simulink model "sgMdl_IO207_DigitalLoopback"  (R2024b)
settings: Solver=FixedStepAuto  StartTime=0.0  StopTime=inf  RelTol=1e-3
undefined symbols (not defined in the file): IO1, IO128, IO64, IO65
libraries: speedgoatlib_IO207 x5
Description:
  | IO207 - Digital Loopback
settings Model: ModifiedByFormat=Speedgoat  Creator=Speedgoat  LastModifiedBy=Speedgoat
settings SolverCC: ConcurrentTasks=on  AlgebraicLoopSolver=TrustRegion  PositivePriorityOrder=on
settings DataIOCC: LimitDataPoints=on  SaveFormat=Array  ReturnWorkspaceOutputs=off
settings OptimizationCC: BlockReduction=off  OptimizeBlockIOStorage=off  BufferReuse=off  ReuseModelBlockBuffer=off  GlobalBufferReuse=off  ExpressionFolding=off  ExpressionDepthLimit=2147483647  LocalBlockOutputs=off  OptimizeDataStoreBuffers=off  BusAssignmentInplaceUpdate=off
settings DebuggingCC: UnderspecifiedInitializationDetection=Classic  MergeDetectMultiDrivingBlocksExec=none  SolverPrmCheckMsg=warning  TasksWithSamePriorityMsg=none  FcnCallInpInsideContextMsg=warning  StateNameClashWarn=warning  SFUnexpectedBacktrackingDiag=warning  SFNoUnconditionalDefaultTransitionDiag=warning  SFExecutionAtInitializationDiag=none  ArithmeticOperatorsInVariantConditions=warning
settings HardwareCC: ProdBitPerLong=64  ProdLongLongMode=on  ProdHWDeviceType=Intel->x86-64 (Linux 64)
settings ModelReferenceCC: EnableRefExpFcnMdlSchedulingChecks=on  PropagateSignalLabelsOutOfModel=off
settings SFSimCC: SimUseLocalCustomCode=off  CustomCodeUndefinedFunction=UseInterfaceOnly
settings RTWCC: Description=Speedgoat Real-Time Target Machine  SystemTargetFile=speedgoat.tlc  TemplateMakefile=slrealtime_default_tmf  RTWUseLocalCustomCode=off  Toolchain=Simulink Real-Time Toolchain  BuildConfiguration=Faster Runs  TargetLang=C++  GPUComputeCapability=3.5  DLArmComputeVersion=19.05
settings CodeAppCC: StateflowObjectComments=on
settings SimulinkRealTimeTargetCC: SubcomponentCodeInterfacePackaging=Reusable function  InstructionSetFMA=off  LogToMDFFile=off  SLRTFileLogMaxRuns=10  UseGCCFastMath=on
settings ConfigComp: CovMetricSettings=dw  CovSaveCumulativeToWorkspaceVar=on  CovSaveSingleToWorkspaceVar=on  CovExternalEMLEnable=off  CovSFcnEnable=off  CovBoundaryAbsTol=1.0e-5

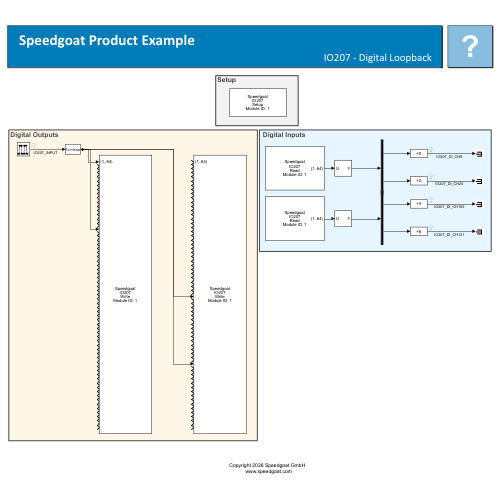
[thumbnail: Simulink's stored preview of the top-level diagram]
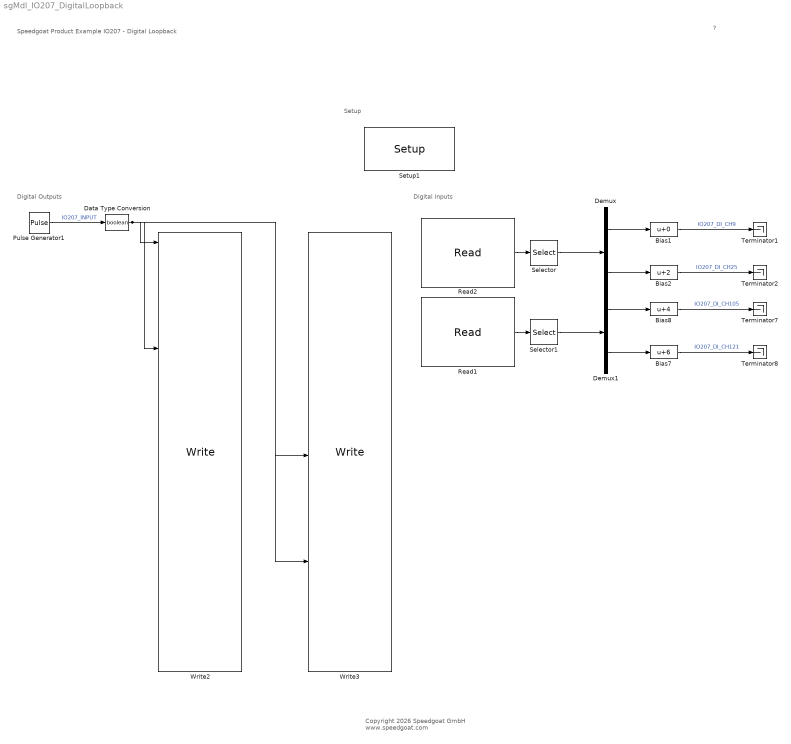
== system sgMdl_IO207_DigitalLoopback ==
  note: Digital Inputs
  note: Digital Outputs
  note: Setup
  note: Speedgoat Product Example
      | IO207 - Digital Loopback
  note: ?
  note: Copyright 2026 Speedgoat GmbH
      |  www.speedgoat.com
  Bias1 : Bias  SaturateOnIntegerOverflow=off
  Bias2 : Bias  Bias=2  SaturateOnIntegerOverflow=off
  Bias7 : Bias  Bias=6  SaturateOnIntegerOverflow=off
  Bias8 : Bias  Bias=4  SaturateOnIntegerOverflow=off
  Data Type Conversion : DataTypeConversion  OutDataTypeStr=boolean  SaturateOnIntegerOverflow=off  RndMeth=Floor
  Demux : Demux  Outputs=2
  Demux1 : Demux  Outputs=2
  Pulse Generator1 : DiscretePulseGenerator  Amplitude=0.8  Period=200  PulseWidth=100  SampleTime=0.001
  Read1 : speedgoatlib_IO207/Read  parModuleId=1  parChannelGroup=Rear  parPortType=1 port with 32 or 64 element vector of type double  parSampleTime=0.001  parPciSlot=-1  parFrontChannelsEn=IO1 ... IO64  parFrontSimuUpdate=OFF  parFrontDirections=[1 0 1 0 1 0 1 0]  parRearChannelsEn=IO65 ... IO128  parRearSimuUpdate=OFF  parRearDirections=[1 0 1 0 1 0 1 0]  parRearDisable=0
      settings: SourceProductName=Simulink Real-Time: Speedgoat I/O Blockset
  Read2 : speedgoatlib_IO207/Read  parModuleId=1  parChannelGroup=Front  parPortType=1 port with 32 or 64 element vector of type double  parSampleTime=0.001  parPciSlot=-1  parFrontChannelsEn=IO1 ... IO64  parFrontSimuUpdate=OFF  parFrontDirections=[1 0 1 0 1 0 1 0]  parRearChannelsEn=IO65 ... IO128  parRearSimuUpdate=OFF  parRearDirections=[1 0 1 0 1 0 1 0]  parRearDisable=0
      settings: SourceProductName=Simulink Real-Time: Speedgoat I/O Blockset
  Selector : Selector  InputPortWidth=64  IndexOptions=Index vector (dialog)  Indices=[9 25]  OutputSizes=1
  Selector1 : Selector  InputPortWidth=64  IndexOptions=Index vector (dialog)  Indices=[105 121]-64  OutputSizes=1
  Setup1 : speedgoatlib_IO207/Setup  parModuleId=1  parPciSlot=-1  parFrontChannelsEn=IO1 ... IO64  parFrontSimuUpdate=OFF  parFrontDirections=[1 0 1 0 1 0 1 0]  parFrontPullResistors=[0]  parFrontInitValues=[0]  parFrontResetValues=[1]  parRearChannelsEn=IO65 ... IO128  parRearSimuUpdate=OFF  parRearDirections=[1 0 1 0 1 0 1 0]  parRearPullResistors=[0]  parRearInitValues=[0]  parRearResetValues=[1]  parRearDisable=off
      settings: SourceProductName=Simulink Real-Time: Speedgoat I/O Blockset
  Terminator{1..2,7..8} (4 alike) : Terminator
  Write2 : speedgoatlib_IO207/Write  parModuleId=1  parChannelGroup=Front  parPortType=32 or 64 ports of type boolean  parSampleTime=-1  parPciSlot=-1  parFrontChannelsEn=IO1 ... IO64  parFrontSimuUpdate=OFF  parFrontDirections=[1 0 1 0 1 0 1 0]  parRearChannelsEn=IO65 ... IO128  parRearSimuUpdate=OFF  parRearDirections=[1 0 1 0 1 0 1 0]  parRearDisable=0
      settings: SourceProductName=Simulink Real-Time: Speedgoat I/O Blockset
  Write3 : speedgoatlib_IO207/Write  parModuleId=1  parChannelGroup=Rear  parPortType=32 or 64 ports of type boolean  parSampleTime=-1  parPciSlot=-1  parFrontChannelsEn=IO1 ... IO64  parFrontSimuUpdate=OFF  parFrontDirections=[1 0 1 0 1 0 1 0]  parRearChannelsEn=IO65 ... IO128  parRearSimuUpdate=OFF  parRearDirections=[1 0 1 0 1 0 1 0]  parRearDisable=0
      settings: SourceProductName=Simulink Real-Time: Speedgoat I/O Blockset
  wires:
  Data Type Conversion/1 -> Write2/17, Write2/1, Write3/33, Write3/49
  Read1/1 -> Selector1/1
  Pulse Generator1/1 -> Data Type Conversion/1  "IO207_INPUT"
  Bias7/1 -> Terminator8/1  "IO207_DI_CH121"
  Selector1/1 -> Demux1/1
  Selector/1 -> Demux/1
  Bias1/1 -> Terminator1/1  "IO207_DI_CH9"
  Bias8/1 -> Terminator7/1  "IO207_DI_CH105"
  Bias2/1 -> Terminator2/1  "IO207_DI_CH25"
  Read2/1 -> Selector/1
  Demux/1 -> Bias1/1
  Demux/2 -> Bias2/1
  Demux1/1 -> Bias8/1
  Demux1/2 -> Bias7/1
